simulink model "Adaptive_MPC_Controller"  (R2024b)
settings: configuration reference "controller_config" (kept outside this file)
undefined symbols (not defined in the file or in its folder): div_min_MPC, I_val, K_f_val, K_r_val, l_f_val, l_r_val, m_val, TimeStep, u0
libraries: mpclib x1
settings Model: DataDictionary=sim_data_vehicle.sldd  Creator=tshintai  LastModifiedBy=tshintai
settings ConfigSetRef: SourceName=controller_config

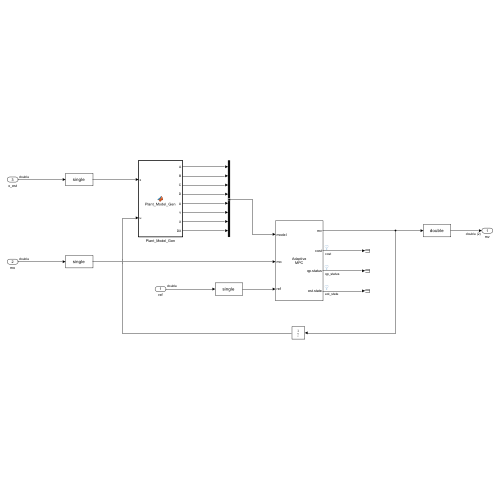
[thumbnail: Simulink's stored preview of the top-level diagram]
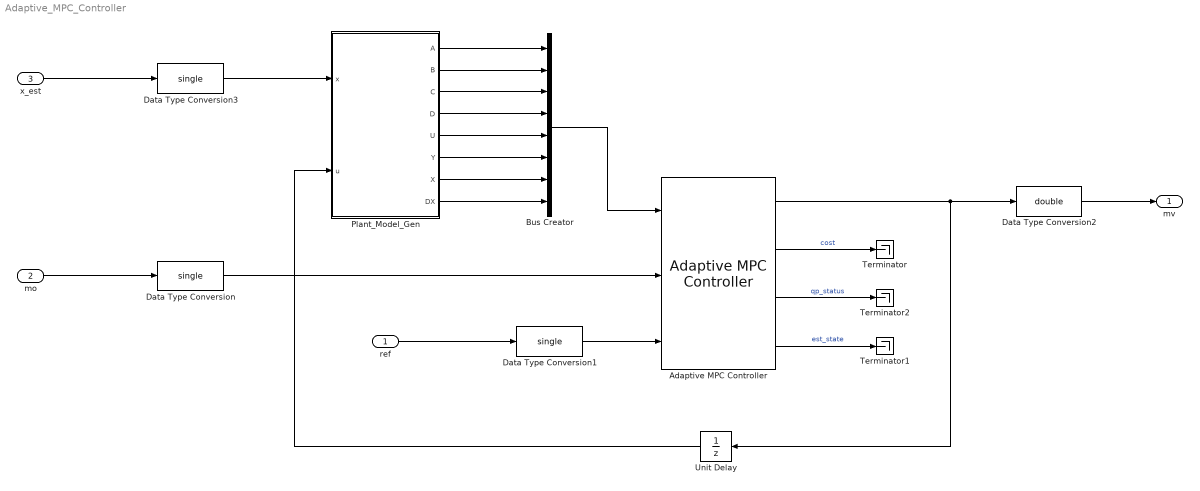
== system Adaptive_MPC_Controller ==
  ref : Inport  OutDataTypeStr=double  PortDimensions=yNum_MPC
  mo : Inport  Port=2  OutDataTypeStr=double  PortDimensions=yNum_MPC
  x_est : Inport  Port=3  OutDataTypeStr=double  PortDimensions=xNum_MPC
  Adaptive MPC Controller : mpclib/Adaptive MPC Controller  SCDEnableBlockLinearizationSpecification=on  mpcobj=mpcObj  enable_value=0  updateMPCinCallerWorkspace=on  md_inport=off  mv_inport=off  uref_inport=off  return_cost=on  return_mvseq=off  return_qpstatus=on  return_xseq=off  return_state=on  return_ovseq=off  state_inport=off  isltv_plant=off  umin_inport=off  umax_inport=off  ymin_inport=off  ymax_inport=off  cc_inport=off  ywt_inport=off  uwt_inport=off  duwt_inport=off  rhoeps_inport=off  pm_inport=off  MaximumP=10  HorizonChoice=FixedHorizon  BlockDataType=single  SampleTimeInherited=off  switch_inport=off
  Bus Creator : BusCreator  Inputs=8
  Data Type Conversion : DataTypeConversion  OutDataTypeStr=single  SaturateOnIntegerOverflow=off  RndMeth=Floor
  Data Type Conversion1 : DataTypeConversion  OutDataTypeStr=single  SaturateOnIntegerOverflow=off  RndMeth=Floor
  Data Type Conversion2 : DataTypeConversion  OutDataTypeStr=double  SaturateOnIntegerOverflow=off  RndMeth=Floor
  Data Type Conversion3 : DataTypeConversion  OutDataTypeStr=single  SaturateOnIntegerOverflow=off  RndMeth=Floor
  Plant_Model_Gen : MATLAB Function  TreatAsAtomicUnit=on
  Terminator : Terminator
  Terminator1 : Terminator
  Terminator2 : Terminator
  Unit Delay : UnitDelay  InitialCondition=u0  SampleTime=-1  HasFrameUpgradeWarning=on
  mv : Outport  OutDataTypeStr=double  PortDimensions=2
  wires:
  Plant_Model_Gen/2(B) -> Bus Creator/2
  Data Type Conversion2/1 -> mv/1
  x_est/1 -> Data Type Conversion3/1
  Data Type Conversion3/1 -> Plant_Model_Gen/1(x)
  Data Type Conversion/1 -> Adaptive MPC Controller/2
  Adaptive MPC Controller/1 -> Data Type Conversion2/1, Unit Delay/1
  Plant_Model_Gen/4(D) -> Bus Creator/4
  Adaptive MPC Controller/3 -> Terminator2/1  "qp_status"
  Plant_Model_Gen/1(A) -> Bus Creator/1
  Plant_Model_Gen/6(Y) -> Bus Creator/6
  Plant_Model_Gen/7(X) -> Bus Creator/7
  mo/1 -> Data Type Conversion/1
  Data Type Conversion1/1 -> Adaptive MPC Controller/3
  ref/1 -> Data Type Conversion1/1
  Plant_Model_Gen/5(U) -> Bus Creator/5
  Bus Creator/1 -> Adaptive MPC Controller/1
  Adaptive MPC Controller/2 -> Terminator/1  "cost"
  Adaptive MPC Controller/4 -> Terminator1/1  "est_state"
  Plant_Model_Gen/3(C) -> Bus Creator/3
  Plant_Model_Gen/8(DX) -> Bus Creator/8
  Unit Delay/1 -> Plant_Model_Gen/2(u)

== matlab function Adaptive_MPC_Controller/Plant_Model_Gen ==
  data: x input; u input; A output size=[xNum_MPC, xNum_MPC]; B output size=[xNum_MPC, uNum_MPC]; C output size=[yNum_MPC, xNum_MPC]; D output size=[yNum_MPC, uNum_MPC]; U output size=[uNum_MPC, 1]; Y output size=[yNum_MPC, 1]; X output size=[xNum_MPC, 1]; DX output size=[xNum_MPC, 1]; TimeStep parameter; I_val parameter; K_f_val parameter; K_r_val parameter; l_f_val parameter; l_r_val parameter; m_val parameter; div_min_MPC parameter
function [A, B, C, D, U, Y, X, DX] = Plant_Model_Gen(x, u, TimeStep,...
    I_val, K_f_val, K_r_val, l_f_val, l_r_val, m_val, div_min_MPC)

ts = cast(TimeStep, 'like', x);

[A, B, C, D, U, Y, X, DX] = calc_Discrete_SS_for_Adaptive( ...
    I_val, K_f_val, K_r_val, l_f_val, l_r_val, m_val, ts, x, u, div_min_MPC);

end
